simulink model "UAV"  (R2025b)
settings: Solver=ode3  StartTime=0.0  StopTime=inf  FixedStep=Sim.Ts_fisica  RelTol=1e-3
PostLoadFcn:
  | Init
InitFcn:
  | Init
model workspace (MAT data in the model file):
  Mass = 1
undefined symbols (not defined in the file): DiscIntNeverNeededParam, Drone, DWORK0, DWORK1, DWORK10, DWORK11, DWORK12, DWORK13, DWORK14, DWORK15, DWORK16, DWORK17, DWORK18, DWORK19, DWORK2, DWORK20, DWORK21, DWORK22, DWORK23, DWORK24, DWORK3, DWORK4, DWORK5, DWORK6, DWORK7, DWORK8, DWORK9, F, Light, MIL, Sim
libraries: simulink x35, slpidlib x11, vrlib x4, aerolibwind2 x2, sim3dlib x2, uavsim3dlib x2
(part 5 of 8)

== system UAV/Flight Controller Software/Flight Controller Software SIL ==
  Pilot Inputs : Inport
  Power_Status : Inport  Port=2
  Measurements_In : Inport  Port=3
  Flight Controller Software_sfcn : S-Function  FunctionName=Flight_sf  SFunctionModules=""  SFunctionDeploymentMode=off  EnableBusSupport=off  SFcnStateName=DWORK0,DWORK1,DWORK2,DWORK3,DWORK4,DWORK5,DWORK6,DWORK7,DWORK8,DWORK9,DWORK10,DWORK11,DWORK12,DWORK13,DWORK14,DWORK15,DWORK16,DWORK17,DWORK18,DWORK19,DWORK20,DWORK21,DWORK22,DWORK23,DWORK24  mask{rtw_sf_name=Flight_sf, showVar=off}
      mask prompts: rtw_sf_name "Simulink:masks:GenSFuncName_MP"; showVar "Simulink:masks:GenSFuncShowModuleList_MP"
      mask help: Simulink:masks:GenSFuncDesc_MD
      mask init:
      | displist = '';
      | if ~strcmp(get_param(gcb, 'FunctionName'), rtw_sf_name);
      |   set_param(gcb, 'FunctionName', rtw_sf_name);
      | end
      | % Check if we are generating code
      | rtw_mode = false;
      | if strcmpi(get_param(bdroot(gcb),'SimulationStatus'),'Initializing')
      | 	rtw_mode = strcmpi(get_param(bdroot(gcb),'BuildingRTWCode'),'on') && ...
      | 		~strcmpi(get_param(bdroot(gcb),'TargetStyle'),'SimulationTarget');
      | end
      | if showVar || rtw_mode
      | 	if exist('rtwsfunc') == 2 | exist('rtwsfunc') == 6
      | 		tmplist = rtwsfunc(rtw_sf_name,gcb);
      | 		tmplist = DAStudio.message('Simulink:masks:GenSFuncListOfModules_IC', tmplist);
      | 	elseif showVar
      | 		tmplist1 = DAStudio.message('Simulink:masks:GenSFuncListOfModules_IC', '');
      |         tmplist2 = DAStudio.message('Simulink:masks:GenSFuncNotLicensed_IC');
      |         tmplist = [tmplist1 tmplist2];
      |  	end
      | end
      | if showVar
      |   displist = tmplist;
      | end
      settings: SFcnIsStateOwnerBlock=on
      settings: CopyFcn=|
      | if ~strcmp(get_param(gcb,'Linkstatus'),'none') && ...
      | ~strcmp(get_param(gcb,'Linkstatus'),'implicit')
      |   set_param(gcb,'LinkStatus','none');
      | end
      mask Help: eval('feval(''rtwprivate'',''rtwhelpview'',''rtw_sfcn_block'')');
      mask Display:
      | port_label('input',1,'Roll');
      | port_label('input',2,'Pitch');
      | port_label('input',3,'Yaw');
      | port_label('input',4,'Throttle');
      | port_label('input',5,'Arm/Disarm');
      | port_label('input',6,'Mode');
      | port_label('input',7,'Volt');
      | port_label('input',8,'Curr');
      | port_label('input',9,'Ve_m');
      | port_label('input',10,'Xe_m');
      | port_label('input',11,'z_m');
      | port_label('input',12,'Mag_m');
      | port_label('input',13,'Wb_m');
      | port_label('input',14,'Acc_m');
      | port_label('output',1,'ALT');
      | port_label('output',2,'VS');
      | port_label('output',3,'SPEED');
      | port_label('output',4,'COMPASS');
      | port_label('output',5,'STATUS');
      | port_label('output',6,'MODE');
      | port_label('output',7,'TIMER');
      | port_label('output',8,'BAT PER');
      | port_label('output',9,'BAT VOLT');
      | port_label('output',10,'PWM_1');
      | port_label('output',11,'PWM_2');
      | port_label('output',12,'PWM_3');
      | port_label('output',13,'PWM_4');
      | port_label('output',14,'PWM_1b');
      | port_label('output',15,'PWM_2b');
      | port_label('output',16,'PWM_3b');
      | port_label('output',17,'PWM_4b');
      | port_label('output',18,'PWM_1a');
      | port_label('output',19,'PWM_2a');
      | port_label('output',20,'PWM_4a');
      | port_label('output',21,'PWM_3a');
      | port_label('output',22,'Vel');
      | port_label('output',23,'Pos');
      | port_label('output',24,'Angles');
      | port_label('output',25,'Rates');
      | port_label('output',26,'System Status');
      | port_label('output',27,'Setpoints');
  __InputSSForSFun__ : Subsystem
  __OutputSSForSFun__ : Subsystem
  "Telemetry " : Outport
  PWM_Out : Outport  Port=2
  FR : Outport  Port=3
  wires:
  Pilot Inputs/1 -> __InputSSForSFun__/1(Pilot Inputs)
  Power_Status/1 -> __InputSSForSFun__/2(Power_Status)
  Measurements_In/1 -> __InputSSForSFun__/3(Measurements_In)
  __InputSSForSFun__/1(__UniqueOutportName__1__) -> Flight Controller Software_sfcn/1
  __InputSSForSFun__/2(__UniqueOutportName__2__) -> Flight Controller Software_sfcn/2
  __InputSSForSFun__/3(__UniqueOutportName__3__) -> Flight Controller Software_sfcn/3
  __InputSSForSFun__/4(__UniqueOutportName__4__) -> Flight Controller Software_sfcn/4
  __InputSSForSFun__/5(__UniqueOutportName__5__) -> Flight Controller Software_sfcn/5
  __InputSSForSFun__/6(__UniqueOutportName__6__) -> Flight Controller Software_sfcn/6
  __InputSSForSFun__/7(__UniqueOutportName__7__) -> Flight Controller Software_sfcn/7
  __InputSSForSFun__/8(__UniqueOutportName__8__) -> Flight Controller Software_sfcn/8
  __InputSSForSFun__/9(__UniqueOutportName__9__) -> Flight Controller Software_sfcn/9
  __InputSSForSFun__/10(__UniqueOutportName__10__) -> Flight Controller Software_sfcn/10
  __InputSSForSFun__/11(__UniqueOutportName__11__) -> Flight Controller Software_sfcn/11
  __InputSSForSFun__/12(__UniqueOutportName__12__) -> Flight Controller Software_sfcn/12
  __InputSSForSFun__/13(__UniqueOutportName__13__) -> Flight Controller Software_sfcn/13
  __InputSSForSFun__/14(__UniqueOutportName__14__) -> Flight Controller Software_sfcn/14
  Flight Controller Software_sfcn/1 -> __OutputSSForSFun__/1(__UniqueInportName__1__)
  Flight Controller Software_sfcn/2 -> __OutputSSForSFun__/2(__UniqueInportName__2__)
  Flight Controller Software_sfcn/3 -> __OutputSSForSFun__/3(__UniqueInportName__3__)
  Flight Controller Software_sfcn/4 -> __OutputSSForSFun__/4(__UniqueInportName__4__)
  Flight Controller Software_sfcn/5 -> __OutputSSForSFun__/5(__UniqueInportName__5__)
  Flight Controller Software_sfcn/6 -> __OutputSSForSFun__/6(__UniqueInportName__6__)
  Flight Controller Software_sfcn/7 -> __OutputSSForSFun__/7(__UniqueInportName__7__)
  Flight Controller Software_sfcn/8 -> __OutputSSForSFun__/8(__UniqueInportName__8__)
  Flight Controller Software_sfcn/9 -> __OutputSSForSFun__/9(__UniqueInportName__9__)
  Flight Controller Software_sfcn/10 -> __OutputSSForSFun__/10(__UniqueInportName__10__)
  Flight Controller Software_sfcn/11 -> __OutputSSForSFun__/11(__UniqueInportName__11__)
  Flight Controller Software_sfcn/12 -> __OutputSSForSFun__/12(__UniqueInportName__12__)
  Flight Controller Software_sfcn/13 -> __OutputSSForSFun__/13(__UniqueInportName__13__)
  Flight Controller Software_sfcn/14 -> __OutputSSForSFun__/14(__UniqueInportName__14__)
  Flight Controller Software_sfcn/15 -> __OutputSSForSFun__/15(__UniqueInportName__15__)
  Flight Controller Software_sfcn/16 -> __OutputSSForSFun__/16(__UniqueInportName__16__)
  Flight Controller Software_sfcn/17 -> __OutputSSForSFun__/17(__UniqueInportName__17__)
  Flight Controller Software_sfcn/18 -> __OutputSSForSFun__/18(__UniqueInportName__18__)
  Flight Controller Software_sfcn/19 -> __OutputSSForSFun__/19(__UniqueInportName__19__)
  Flight Controller Software_sfcn/20 -> __OutputSSForSFun__/20(__UniqueInportName__20__)
  Flight Controller Software_sfcn/21 -> __OutputSSForSFun__/21(__UniqueInportName__21__)
  Flight Controller Software_sfcn/22 -> __OutputSSForSFun__/22(__UniqueInportName__22__)
  Flight Controller Software_sfcn/23 -> __OutputSSForSFun__/23(__UniqueInportName__23__)
  Flight Controller Software_sfcn/24 -> __OutputSSForSFun__/24(__UniqueInportName__24__)
  Flight Controller Software_sfcn/25 -> __OutputSSForSFun__/25(__UniqueInportName__25__)
  Flight Controller Software_sfcn/26 -> __OutputSSForSFun__/26(__UniqueInportName__26__)
  Flight Controller Software_sfcn/27 -> __OutputSSForSFun__/27(__UniqueInportName__27__)
  __OutputSSForSFun__/1("Telemetry ") -> "Telemetry "/1
  __OutputSSForSFun__/2(PWM_Out) -> PWM_Out/1
  __OutputSSForSFun__/3(FR) -> FR/1

== system UAV/Pilot Interface/Real_Receiver_Driver  ==
  Telemetry : Inport
  Command Acquisition : Subsystem
  Flight Data Display : Subsystem
  Pilot Inputs : Outport
  wires:
  Command Acquisition/1(Pilot Inputs) -> Pilot Inputs/1
  Telemetry/1 -> Flight Data Display/1(Telemetry)

== system UAV/Pilot Interface/SIM_Flightstick_HotasX56  ==
  Telemetry : Inport
  Command Acquisition : Subsystem
  Flight Data Display : Subsystem
  Pilot Inputs : Outport
  wires:
  Command Acquisition/1(Pilot Inputs) -> Pilot Inputs/1
  Telemetry/1 -> Flight Data Display/1(Telemetry)

== system UAV/Vehicle Interface/Real_Hardware_Drivers ==
  PWM_In : Inport
  FR : Inport  Port=2
  ADC : Subsystem
  Actuators : Subsystem
  Battery : Subsystem
  Body Dynamics : Subsystem
  Bus Creator : BusCreator  Inputs=6
  Bus Creator1 : BusCreator  Inputs=2
  Bus Creator2 : BusCreator  Inputs=2
  Bus Creator3 : BusCreator  Inputs=4
  Bus Selector : BusSelector  OutputSignals=PWM_1,PWM_2,PWM_3,PWM_4
  Bus Selector1 : BusSelector  OutputSignals=Nav_Data,Pid_Effort,PWM_Motors
  ESC_Quantization_Model : Subsystem
  Flight Recorder : Subsystem
  Sensors : Subsystem
  To Workspace : ToWorkspace  VariableName=Ground_Truth  SaveFormat=Structure With Time  SampleTime=-1
  To Workspace1 : ToWorkspace  VariableName=Measurements  SaveFormat=Structure With Time  SampleTime=-1
  Visualization : Subsystem
  Measurements_Out : Outport
  Battery_Parameters : Outport  Port=2
  wires:
  Actuators/1(M1) -> Body Dynamics/1(F1)
  Actuators/2(M2) -> Body Dynamics/2(F2)
  Actuators/3(M3) -> Body Dynamics/3(F3)
  Actuators/4(M4) -> Body Dynamics/4(F4)
  Body Dynamics/1(Ve_gt) -> Sensors/1(Ve)
  Body Dynamics/2(Xe_gt) -> Sensors/2(Xe), Bus Creator1/1  "Xe_gt"
  Body Dynamics/3(Euler_gt) -> Sensors/3(Euler), Bus Creator1/2  "Euler_gt"
  Body Dynamics/4(DCMbe) -> Sensors/4(DCMbe)
  Body Dynamics/6(Wb_gt) -> Sensors/6(Wb)
  Sensors/1(Ve_m) -> Bus Creator/1  "Ve_m"
  Bus Creator/1 -> To Workspace1/1, Measurements_Out/1
  PWM_In/1 -> Bus Selector/1
  Bus Selector/1 -> Battery/1(PWM_1), Actuators/1(PWM_1)  "<PWM_1>"
  Bus Selector/2 -> Battery/2(PWM_2), Actuators/2(PWM_2)  "<PWM_2>"
  Bus Selector/3 -> Battery/3(PWM_3), Actuators/3(PWM_3)  "<PWM_3>"
  Bus Selector/4 -> Battery/4(PWM_4), Actuators/4(PWM_4)  "<PWM_4>"
  Bus Creator1/1 -> Visualization/1(Ground Truth)
  Body Dynamics/5(Vb_gt) -> Sensors/5(Vb)
  Sensors/2(Xe_m) -> Bus Creator/2  "Xe_m"
  Sensors/3(z_m) -> Bus Creator/3  "z_m"
  Sensors/4(Mag_m) -> Bus Creator/4  "Mag_m"
  Battery/1(Battery_Volt) -> ADC/1(In1)
  ADC/1(Out1) -> Bus Creator2/1  "Volt"
  Bus Creator2/1 -> Battery_Parameters/1
  Battery/2(Battery_Curr) -> ADC/2(Battery_Curr)
  ADC/2(Out2) -> Bus Creator2/2  "Curr"
  FR/1 -> Bus Selector1/1
  Bus Selector1/1 -> Flight Recorder/1(Nav_Data)  "<Nav_Data>"
  Bus Selector1/2 -> Flight Recorder/2(PID_Effort)  "<Pid_Effort>"
  Bus Selector1/3 -> Flight Recorder/3(Motor_PWM)  "<PWM_Motors>"
  Sensors/7("Euler_gt ") -> Bus Creator3/1  "Euler_gt"
  Sensors/8("Vb_gt ") -> Bus Creator3/2  "Vb_gt"
  Sensors/9(Xe_gt) -> Bus Creator3/3  "Xe_gt"
  Sensors/10(Ve_gt) -> Bus Creator3/4  "Ve_gt"
  Bus Creator3/1 -> To Workspace/1
  Sensors/5(Gyro_m) -> Bus Creator/5  "Wb_m"
  Sensors/6(Acc_m) -> Bus Creator/6  "Acc_m"

== system UAV/Vehicle Interface/Sim_Plant_Model ==
  PWM_In : Inport
  FR : Inport  Port=2
  ADC : Subsystem
  Actuators : Subsystem
  Battery : Subsystem
  Body Dynamics : Subsystem
  Bus Creator : BusCreator  Inputs=6
  Bus Creator1 : BusCreator  Inputs=2
  Bus Creator2 : BusCreator  Inputs=2
  Bus Creator3 : BusCreator  Inputs=4
  Bus Selector : BusSelector  OutputSignals=PWM_1,PWM_2,PWM_3,PWM_4
  Bus Selector1 : BusSelector  OutputSignals=Nav_Data,Pid_Effort,PWM_Motors
  ESC_Quantization_Model : Subsystem
  Flight Recorder : Subsystem
  Sensors : Subsystem
  To Workspace : ToWorkspace  VariableName=Ground_Truth  SaveFormat=Structure With Time  SampleTime=-1
  To Workspace1 : ToWorkspace  VariableName=Measurements  SaveFormat=Structure With Time  SampleTime=-1
  Visualization : Subsystem
  Measurements_Out : Outport
  Battery_Parameters : Outport  Port=2
  wires:
  Actuators/1(M1) -> Body Dynamics/1(F1)
  Actuators/2(M2) -> Body Dynamics/2(F2)
  Actuators/3(M3) -> Body Dynamics/3(F3)
  Actuators/4(M4) -> Body Dynamics/4(F4)
  Body Dynamics/1(Ve_gt) -> Sensors/1(Ve)
  Body Dynamics/2(Xe_gt) -> Sensors/2(Xe), Bus Creator1/1  "Xe_gt"
  Body Dynamics/3(Euler_gt) -> Sensors/3(Euler), Bus Creator1/2  "Euler_gt"
  Body Dynamics/4(DCMbe) -> Sensors/4(DCMbe)
  Body Dynamics/6(Wb_gt) -> Sensors/6(Wb)
  Sensors/1(Ve_m) -> Bus Creator/1  "Ve_m"
  Bus Creator/1 -> To Workspace1/1, Measurements_Out/1
  PWM_In/1 -> Bus Selector/1
  Bus Selector/1 -> Battery/1(PWM_1), Actuators/1(PWM_1)  "<PWM_1>"
  Bus Selector/2 -> Battery/2(PWM_2), Actuators/2(PWM_2)  "<PWM_2>"
  Bus Selector/3 -> Battery/3(PWM_3), Actuators/3(PWM_3)  "<PWM_3>"
  Bus Selector/4 -> Battery/4(PWM_4), Actuators/4(PWM_4)  "<PWM_4>"
  Bus Creator1/1 -> Visualization/1(Ground Truth)
  Body Dynamics/5(Vb_gt) -> Sensors/5(Vb)
  Sensors/2(Xe_m) -> Bus Creator/2  "Xe_m"
  Sensors/3(z_m) -> Bus Creator/3  "z_m"
  Sensors/4(Mag_m) -> Bus Creator/4  "Mag_m"
  Battery/1(Battery_Volt) -> ADC/1(In1)
  ADC/1(Out1) -> Bus Creator2/1  "Volt"
  Bus Creator2/1 -> Battery_Parameters/1
  Battery/2(Battery_Curr) -> ADC/2(Battery_Curr)
  ADC/2(Out2) -> Bus Creator2/2  "Curr"
  FR/1 -> Bus Selector1/1
  Bus Selector1/1 -> Flight Recorder/1(Nav_Data)  "<Nav_Data>"
  Bus Selector1/2 -> Flight Recorder/2(PID_Effort)  "<Pid_Effort>"
  Bus Selector1/3 -> Flight Recorder/3(Motor_PWM)  "<PWM_Motors>"
  Sensors/7("Euler_gt ") -> Bus Creator3/1  "Euler_gt"
  Sensors/8("Vb_gt ") -> Bus Creator3/2  "Vb_gt"
  Sensors/9(Xe_gt) -> Bus Creator3/3  "Xe_gt"
  Sensors/10(Ve_gt) -> Bus Creator3/4  "Ve_gt"
  Bus Creator3/1 -> To Workspace/1
  Sensors/5(Gyro_m) -> Bus Creator/5  "Wb_m"
  Sensors/6(Acc_m) -> Bus Creator/6  "Acc_m"
